simulink model "simulator_maats_wrench"  (R2025b)
settings: Solver=ode8  StartTime=0.0  StopTime=3  FixedStep=1e-4  RelTol=1e-3
values from neighbouring files (symbols this model uses):
  att_ctrl = struct    [parametrosCarga4x.m]
  cable = struct    [parametrosCarga4x.m]
  payload = struct    [parametrosCarga4x.m]
  pos_ctrl = struct    [parametrosCarga4x.m]
  uav1 = uav    [parametrosCarga4x.m]
  uav2 = uav    [parametrosCarga4x.m]
libraries: ASK x2
settings Model: Creator=ateveraz  LastModifiedBy=ateveraz
settings DebuggingCC: AlgebraicLoopMsg=none

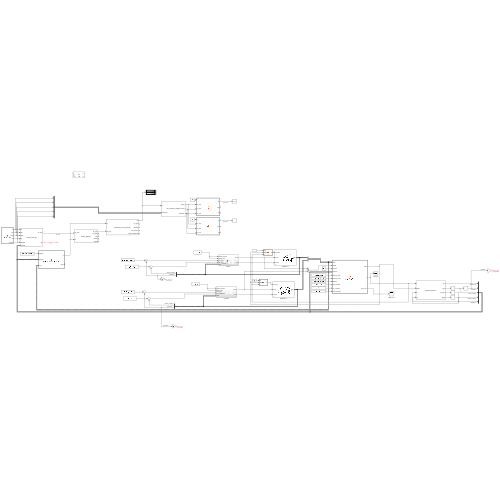
[thumbnail: Simulink's stored preview of the top-level diagram]
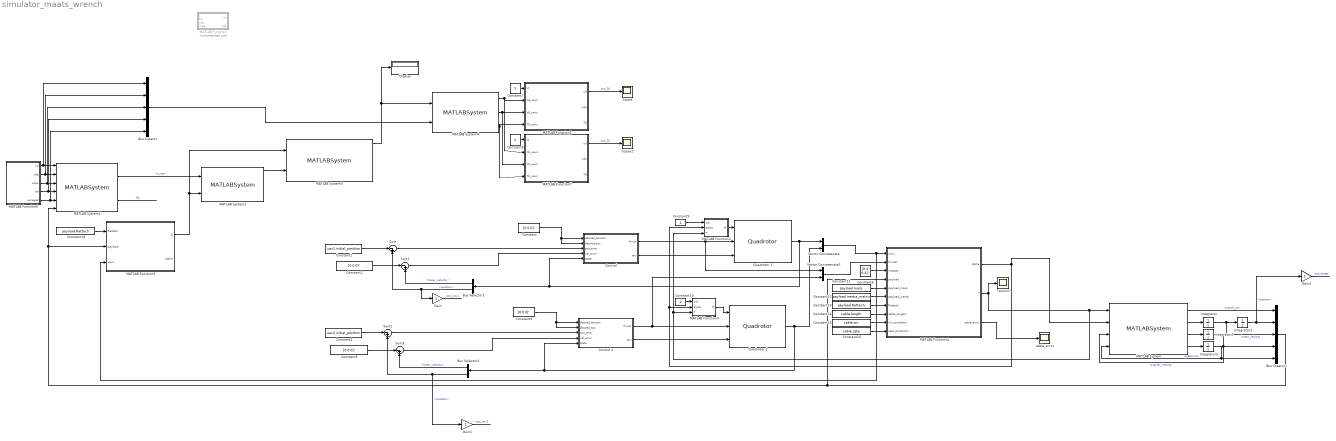
== system simulator_maats_wrench ==
  Bus Creator : BusCreator  Inputs=5  OutDataTypeStr=Bus: payload_reference
      settings: InheritFromInputs=off
  Bus Creator1 : BusCreator  Inputs=5  OutDataTypeStr=Bus: payload_state  NonVirtualBus=on
  Bus Selector1 : BusSelector  OutputSignals=linear_velocity,position
  Bus Selector2 : BusSelector  OutputSignals=linear_velocity,position
  Constant{,2..3,5} (4 alike) : Constant  Value=[0 0 0]'
  Constant1 : Constant  Value=uav1.initial_position
  Constant10 : Constant  Value=2
  Constant11 : Constant  Value=payload.mass
  Constant12 : Constant  Value=payload.inertia_matrix
  Constant13 : Constant  Value=payload.Rattach
  Constant14 : Constant  Value=cable.length
  Constant15 : Constant  Value=cable.wn
  Constant16 : Constant  Value=cable.zeta
  Constant18 : Constant  Value=payload.Rattach
  Constant4 : Constant  Value=uav2.initial_position
  Constant6 : Constant  Value=[0.4 0.4]'
  Constant7 : Constant
  Constant8 : Constant  Value=2
  Constant9 : Constant
  Control : Subsystem
  Control 2 : Subsystem
  Display : Display
  Gain : Gain
  Gain1 : Gain
  Gain2 : Gain
  Integrator : Integrator  InitialCondition=payload.initial_linear_velocity
  Integrator1 : Integrator  InitialCondition=payload.initial_position
  Integrator2 : Integrator  InitialCondition=payload.initial_angular_velocity
  Integrator3 : Integrator  InitialCondition=payload.initial_quaternion
  MATLAB Function : MATLAB Function  Commented=on  TreatAsAtomicUnit=on
  MATLAB Function1 : MATLAB Function  TreatAsAtomicUnit=on
  MATLAB Function2 : MATLAB Function  TreatAsAtomicUnit=on
  MATLAB Function3 : MATLAB Function  TreatAsAtomicUnit=on
  MATLAB Function4 : MATLAB Function  TreatAsAtomicUnit=on
  MATLAB Function5 : MATLAB Function  TreatAsAtomicUnit=on
  MATLAB Function6 : MATLAB Function  TreatAsAtomicUnit=on
  MATLAB Function7 : MATLAB Function  TreatAsAtomicUnit=on
  MATLAB System : MATLABSystem  System=payload_dynamics  mass=payload.mass  inertia_matrix=payload.inertia_matrix  Rattach=payload.Rattach  N=payload.number_uav  SimulateUsing=Code generation
      mask Type: payload_dynamics
  MATLAB System1 : MATLABSystem  System=nominal_controller  mass=0.225  Ks=diag( [ 0, 0, 4.0, 0, 0.25, 0 ] )  Lambda_x=diag( [ 0, 0, 1.5 ] )  Lambda_R=diag( [ 0, 2.0, 0 ] )  SimulateUsing=Interpreted execution
      mask Type: nominal_controller
  MATLAB System2 : MATLABSystem  System=wrench_projector  N=2  RankTolerance=1e-8  SimulateUsing=Interpreted execution
      mask Type: wrench_projector
  MATLAB System3 : MATLABSystem  System=geometric_tension_allocator  N=2  ConditioningThreshold=1e-9  SimulateUsing=Code generation
      mask Type: geometric_tension_allocator
  MATLAB System4 : MATLABSystem  System=uav_reference_regulator  N=2  Rattach=[ 0.5, -0.5; 0, 0; 0, 0 ]  CableLengths=[ 0.8; 0.8 ]  Alpha_d=[ 0, 0; 0, 0; 1, 1 ]  SimulateUsing=Interpreted execution
      mask Type: uav_reference_regulator
  Quadrotor 1 : ASK/Quadrotor  mass=uav1.mass  inertia_matrix=uav1.inertia_matrix  pos0=uav1.initial_position  vel0=uav1.initial_linear_velocity  omega0=uav1.initial_angular_velocity  quat0=uav1.initial_quaternion
      settings: SourceProductName=ASK
  Quadrotor 2 : ASK/Quadrotor  mass=uav2.mass  inertia_matrix=uav2.inertia_matrix  pos0=uav2.initial_position  vel0=uav2.initial_linear_velocity  omega0=uav2.initial_angular_velocity  quat0=uav2.initial_quaternion
      settings: SourceProductName=ASK
  Scope : Scope
      settings: ActiveDisplayYMinimum=-1  ActiveDisplayYMaximum=1  DataLoggingVariableName=ScopeData2
  Scope1 : Scope
      settings: ActiveDisplayYMinimum=-0.9625  ActiveDisplayYMaximum=0.6625  DataLoggingVariableName=ScopeData3
  Sum{,1..3} (4 alike) : Sum  Inputs=|-+
  Tension : Scope
      settings: ActiveDisplayYMinimum=0.78222189935535491  ActiveDisplayYMaximum=1.5736614423871715
  Vector Concatenate : Concatenate
  Vector Concatenate1 : Concatenate
  cable_error : Scope
      settings: ActiveDisplayYMinimum=-0.0074413173902670993  ActiveDisplayYMaximum=0.010827713169143105
  wires:
  Bus Selector1/2 -> Gain/1, Sum/2  "<position>"
  Bus Selector1/1 -> Sum1/2  "<linear_velocity>"
  Quadrotor 1/1 -> Vector Concatenate/1, Control/5(state), Bus Selector1/1
  Sum/1 -> Control/3(pos_error)
  Sum1/1 -> Control/4(vel_error)
  Constant/1 -> Control/1(desired_tension), Control/2(desired_acc)
  Constant2/1 -> Sum1/1
  Control 2/1(thrust) -> Vector Concatenate1/2, Quadrotor 2/2
  MATLAB System/2 -> Integrator/1
  Integrator/1 -> Integrator1/1, Bus Creator1/3  "linear_velocity"
  MATLAB System/3 -> Integrator2/1
  MATLAB System/4 -> Integrator3/1
  Integrator3/1 -> Bus Creator1/5, MATLAB System/4  "quaternion"
  Integrator2/1 -> Bus Creator1/4, MATLAB System/3  "angular_velocity"
  MATLAB System/1 -> Bus Creator1/1  "wrench_ctrl"
  Constant5/1 -> Sum3/1
  Constant3/1 -> Control 2/2(desired_acc), Control 2/1(desired_tension)
  Sum3/1 -> Control 2/4(vel_error)
  Sum2/1 -> Control 2/3(pos_error)
  Quadrotor 2/1 -> Bus Selector2/1, Control 2/5(state), Vector Concatenate/2
  Bus Selector2/1 -> Sum3/2  "<linear_velocity>"
  Vector Concatenate/1 -> MATLAB Function4/1(uavs), MATLAB Function5/3(uavs)
  Vector Concatenate1/1 -> MATLAB Function4/2(thrusts)
  Constant6/1 -> MATLAB Function4/3(masses)
  MATLAB Function4/2(T) -> MATLAB Function3/3(T), MATLAB Function2/3(T), MATLAB System/1, Tension/1
  MATLAB Function4/1(Alpha) -> MATLAB Function3/2(alpha), MATLAB Function2/2(alpha), MATLAB System/2
  Constant9/1 -> MATLAB Function2/1(ind)
  MATLAB Function2/1(tf) -> Quadrotor 1/1
  MATLAB Function3/1(tf) -> Quadrotor 2/1
  Constant10/1 -> MATLAB Function3/1(ind)
  Constant11/1 -> MATLAB Function4/5(payload_mass)
  Constant12/1 -> MATLAB Function4/6(payload_inertia)
  Constant13/1 -> MATLAB Function4/7(Rattach)
  Constant14/1 -> MATLAB Function4/8(cable_lengths)
  Constant15/1 -> MATLAB Function4/9(wn_constraint)
  Constant16/1 -> MATLAB Function4/10(zeta_constraint)
  MATLAB Function4/3(cable_error) -> cable_error/1
  Control/2(tau) -> Quadrotor 1/3
  Control 2/2(tau) -> Quadrotor 2/3
  Control/1(thrust) -> Vector Concatenate1/1, Quadrotor 1/2
  Constant18/1 -> MATLAB Function5/1(Rattach)
  Bus Creator1/1 -> MATLAB Function4/4(payload), MATLAB System1/6, MATLAB Function5/2(payload)
  MATLAB Function6/2(xdp) -> Bus Creator/2, MATLAB System1/2
  MATLAB Function6/3(xdpp) -> Bus Creator/3, MATLAB System1/3
  MATLAB Function6/1(xd) -> Bus Creator/1, MATLAB System1/1
  MATLAB Function6/4(qd) -> Bus Creator/4, MATLAB System1/4
  MATLAB Function6/5(omegad) -> Bus Creator/5, MATLAB System1/5
  MATLAB System1/2 -> ?  "Sp"
  MATLAB System1/1 -> MATLAB System2/1  "wc_raw"
  MATLAB Function5/1(G) -> MATLAB System3/1, MATLAB System2/2
  MATLAB System2/1 -> MATLAB System3/2
  MATLAB System3/1 -> MATLAB System4/1, Display/1
  Bus Creator/1 -> MATLAB System4/2
  Constant7/1 -> MATLAB Function1/1(id)
  MATLAB System4/3 -> MATLAB Function7/4(Td_uavs), MATLAB Function1/4(Td_uavs)
  MATLAB Function1/1(xd) -> Scope/1  "pos_D1"
  MATLAB System4/2 -> MATLAB Function7/3(Vd_uavs), MATLAB Function1/3(Vd_uavs)
  MATLAB System4/1 -> MATLAB Function7/2(Xd_uavs), MATLAB Function1/2(Xd_uavs)
  Constant8/1 -> MATLAB Function7/1(id)
  Constant4/1 -> Sum2/1
  MATLAB Function7/1(xd) -> Scope1/1  "pos_D2"
  Gain/1 -> ?  "pos_uav1"
  Gain1/1 -> ?  "pos_uav2"
  Bus Selector2/2 -> Gain1/1, Sum2/2  "<position>"
  Gain2/1 -> ?  "pos_carga"
  Integrator1/1 -> Gain2/1, Bus Creator1/2  "<position>"
  Constant1/1 -> Sum/1

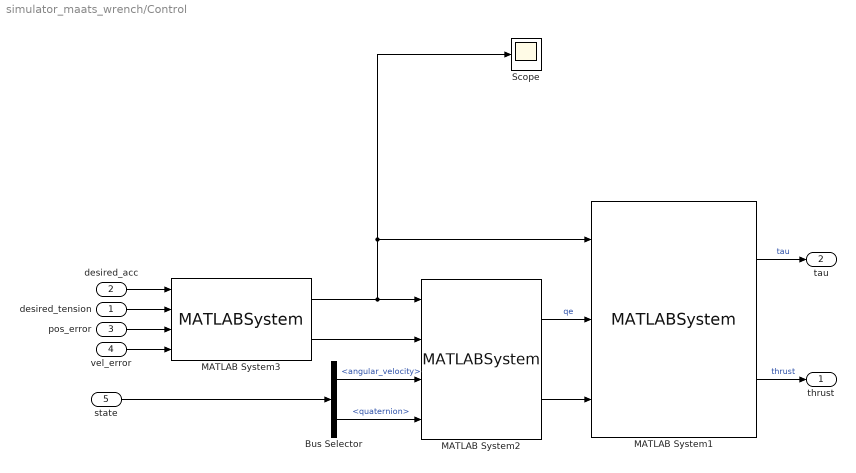
== system simulator_maats_wrench/Control ==
  desired_tension : Inport
  desired_acc : Inport  Port=2
  pos_error : Inport  Port=3
  vel_error : Inport  Port=4
  state : Inport  Port=5
  Bus Selector : BusSelector  OutputSignals=angular_velocity,quaternion
  MATLAB System1 : MATLABSystem  System=AttitudeController  Kd=att_ctrl.Kd  beta=att_ctrl.beta  gamma=att_ctrl.gamma  rho=att_ctrl.rho  SimulateUsing=Code generation
      mask Type: AttitudeController
  MATLAB System2 : MATLABSystem  System=DesiredAttitude  SimulateUsing=Code generation
      mask Type: DesiredAttitude
  MATLAB System3 : MATLABSystem  System=PositionController  Kd=pos_ctrl.Kd  alpha=pos_ctrl.alpha  mass=pos_ctrl.mass  SimulateUsing=Interpreted execution
      mask Type: PositionController
  Scope : Scope
      settings: ActiveDisplayYMinimum=-1  ActiveDisplayYMaximum=1  DataLoggingVariableName=ScopeData4
  thrust : Outport
  tau : Outport  Port=2
  wires:
  MATLAB System2/2 -> MATLAB System1/3
  MATLAB System2/1 -> MATLAB System1/2  "qe"
  Bus Selector/1 -> MATLAB System2/3  "<angular_velocity>"
  Bus Selector/2 -> MATLAB System2/4  "<quaternion>"
  MATLAB System3/2 -> MATLAB System2/2
  state/1 -> Bus Selector/1
  MATLAB System3/1 -> Scope/1, MATLAB System1/1, MATLAB System2/1
  pos_error/1 -> MATLAB System3/3
  vel_error/1 -> MATLAB System3/4
  desired_tension/1 -> MATLAB System3/2
  desired_acc/1 -> MATLAB System3/1
  MATLAB System1/1 -> tau/1  "tau"
  MATLAB System1/2 -> thrust/1  "thrust"

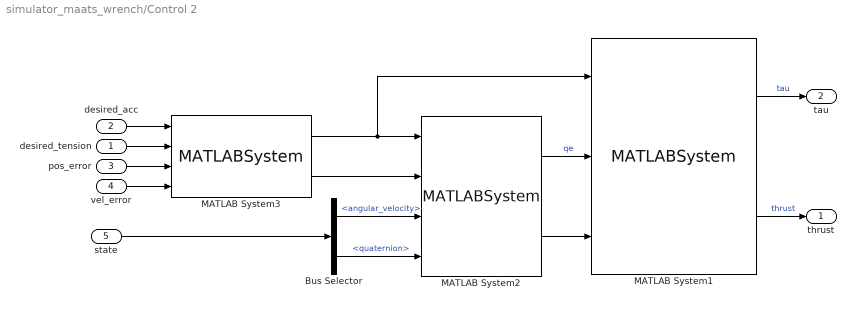
== system simulator_maats_wrench/Control 2 ==
  desired_tension : Inport
  desired_acc : Inport  Port=2
  pos_error : Inport  Port=3
  vel_error : Inport  Port=4
  state : Inport  Port=5
  Bus Selector : BusSelector  OutputSignals=angular_velocity,quaternion
  MATLAB System1 : MATLABSystem  System=AttitudeController  Kd=att_ctrl.Kd  beta=att_ctrl.beta  gamma=att_ctrl.gamma  rho=att_ctrl.rho  SimulateUsing=Code generation
      mask Type: AttitudeController
  MATLAB System2 : MATLABSystem  System=DesiredAttitude  SimulateUsing=Code generation
      mask Type: DesiredAttitude
  MATLAB System3 : MATLABSystem  System=PositionController  Kd=pos_ctrl.Kd  alpha=pos_ctrl.alpha  mass=pos_ctrl.mass  SimulateUsing=Interpreted execution
      mask Type: PositionController
  thrust : Outport
  tau : Outport  Port=2
  wires:
  MATLAB System1/2 -> thrust/1  "thrust"
  MATLAB System1/1 -> tau/1  "tau"
  desired_acc/1 -> MATLAB System3/1
  desired_tension/1 -> MATLAB System3/2
  vel_error/1 -> MATLAB System3/4
  pos_error/1 -> MATLAB System3/3
  MATLAB System3/1 -> MATLAB System2/1, MATLAB System1/1
  state/1 -> Bus Selector/1
  MATLAB System3/2 -> MATLAB System2/2
  Bus Selector/2 -> MATLAB System2/4  "<quaternion>"
  Bus Selector/1 -> MATLAB System2/3  "<angular_velocity>"
  MATLAB System2/1 -> MATLAB System1/2  "qe"
  MATLAB System2/2 -> MATLAB System1/3

== matlab function simulator_maats_wrench/MATLAB Function5 ==
  data: Rattach input; payload input; uavs input; G output; Alpha output
function [G, Alpha] = compute_cable_wrench_map(Rattach, payload, uavs)
    [G, Alpha] = build_cable_wrench_matrix(Rattach, payload, uavs);
end

== matlab function simulator_maats_wrench/MATLAB Function ==
  data: L input; xd output; Td input; xLd input; xLdp input; xdp output
function [xd, xdp] = fcn(L,  Td, xLd, xLdp)
    alpha = zeros(3,1);
    if (norm(Td)~=0)
        alpha = Td/norm(Td);
    end
    xd = xLd - L*alpha;
    xdp = xLdp;
end

== matlab function simulator_maats_wrench/MATLAB Function1 ==
  data: id input; Xd_uavs input; xd output; Vd_uavs input; xdp output; Td output; Td_uavs input
function [xd, xdp, Td] = fcn(id, Xd_uavs, Vd_uavs, Td_uavs)
    xd  = Xd_uavs(:,id);
    xdp = Vd_uavs(:,id);
    Td  = Td_uavs(:,id);
end

== matlab function simulator_maats_wrench/MATLAB Function2 ==
  data: ind input; alpha input; tf output; T input
function tf = fcn(ind, alpha, T)
    tf = - T(ind) * alpha(:, ind);
end

== matlab function simulator_maats_wrench/MATLAB Function3 ==
  data: ind input; alpha input; tf output; T input
function tf = fcn(ind, alpha, T)
    tf = - T(ind) * alpha(:, ind);
end

== matlab function simulator_maats_wrench/MATLAB Function7 ==
  data: id input; Xd_uavs input; xd output; Vd_uavs input; xdp output; Td output; Td_uavs input
function [xd, xdp, Td] = fcn(id, Xd_uavs, Vd_uavs, Td_uavs)
    xd  = Xd_uavs(:,id);
    xdp = Vd_uavs(:,id);
    Td  =  Td_uavs(:,id);
end

== matlab function simulator_maats_wrench/MATLAB Function4 ==
  data: uavs input; Alpha output; thrusts input; masses input; payload input; payload_mass input; payload_inertia input; Rattach input; cable_lengths input; wn_constraint input; zeta_constraint input; T output; cable_error output
function [Alpha, T, cable_error] = rigid_cable_states( ...
    uavs, thrusts, masses, payload, ...
    payload_mass, payload_inertia, Rattach, cable_lengths, ...
    wn_constraint, zeta_constraint)

    [Alpha, T, cable_error] = tensionSolver( uavs, thrusts, masses, payload, payload_mass, payload_inertia, Rattach, cable_lengths, wn_constraint, zeta_constraint);

end

== matlab function simulator_maats_wrench/MATLAB Function6 ==
  data: xd output; xdp output; xdpp output; qd output; omegad output
function [xd, xdp, xdpp, qd, omegad] = regulation
    % Cartesian desired position
    xd   = [0 0 0]';
    xdp  = [0 0 0]';
    xdpp = [0 0 0]';
    % Quaternion-based desired attitude
    qd   = [1 0 0 0]';
    omegad = [0 0 0]';
end
